simulink model "PI_5-67"  (R2025a)
settings: Solver=VariableStepAuto  StartTime=0.0  StopTime=10.0  RelTol=1e-3
values from neighbouring files (symbols this model uses):
  alpha = a    (= 20.6731)    [Rocky_5_closed_loop_poles.m]    (also in Rocky_67.m = a; pole5.m = a)
  beta = b    (= 0.001719)    [Rocky_5_closed_loop_poles.m]    (also in Rocky_67.m = b; pole5.m = b)
  dist_duration = .1    (= 0.1)    [Rocky_5_closed_loop_poles.m]    (also in Rocky_67.m; pole5.m)
  dist_magnitude = pi()/18    [Rocky_5_closed_loop_poles.m]    (also in Rocky_67.m; pole5.m)
  dist_time = 1    [Rocky_5_closed_loop_poles.m]    (also in Rocky_67.m; pole5.m)
  Ki = double(solutions.Ki)    [Rocky_5_closed_loop_poles.m]    (also in Rocky_67.m = (leff / (alpha * beta)) * (alpha^3 / 27 + alpha * omega_n^2); Rocky_closed_loop_poles_23.m; pole5.m = 16528)
  Kp = double(solutions.Kp)    [Rocky_5_closed_loop_poles.m]    (also in Rocky_67.m = (leff / (alpha * beta)) * (alpha^2 / 3 + omega_n^2); Rocky_closed_loop_poles_23.m; pole5.m = 3507.2)
  leff = l    (= 0.4452)    [Rocky_5_closed_loop_poles.m]    (also in Rocky_67.m = L; pole5.m = l)
  omega_n = 4.6939    [Rocky_5_closed_loop_poles.m]    (also in Rocky_67.m = omega_d / sqrt(1 - zeta^2); pole5.m)
  theta_r = 0    [Rocky_5_closed_loop_poles.m]    (also in Rocky_67.m; pole5.m)
libraries: slpidlib x1
settings Model: Creator=nbanse  LastModifiedBy=nbanse

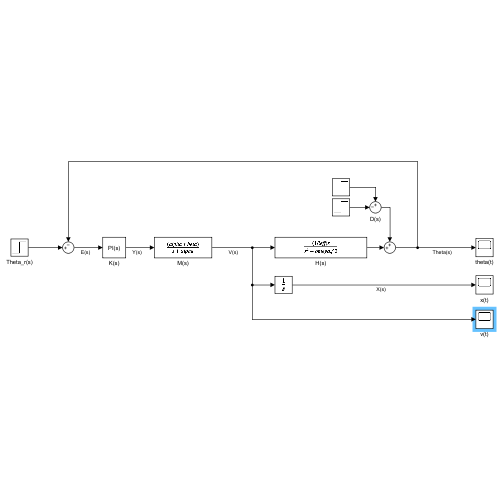
[thumbnail: Simulink's stored preview of the top-level diagram]
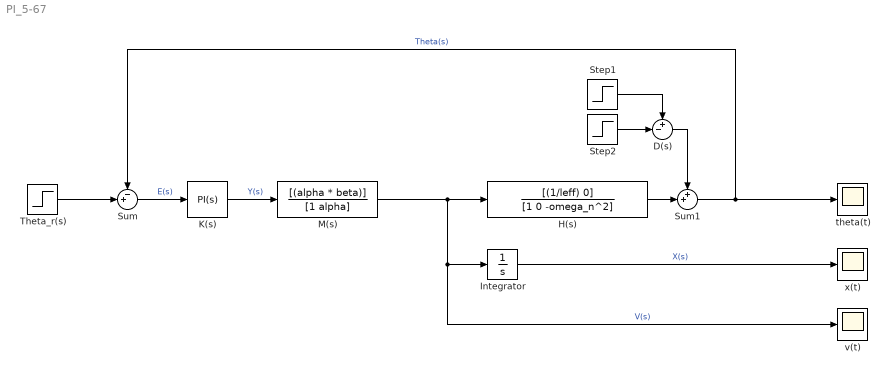
== system PI_5-67 ==
  D(s) : Sum  Inputs=+-|
  H(s) : TransferFcn  Numerator=[(1/leff) 0]  Denominator=[1 0 -omega_n^2]
  Integrator : Integrator
  K(s) : slpidlib/PID Controller  Controller=PI  Form=Parallel  TimeDomain=Continuous-time  UseExternalTs=off  SampleTime=-1  IntegratorMethod=Forward Euler  FilterMethod=Forward Euler  ControllerParametersSource=internal  P=Kp  I=Ki  UseKiTs=off  D=0  UseExternalDerivativeSource=off  N=100  UseFilter=on  TunerSelectOption=Transfer Function Based (PID Tuner App)  InitialConditionSource=internal  InitialConditionForIntegrator=0  InitialConditionForFilter=0  DifferentiatorICPrevScaledInput=0  ExternalReset=none  TrackingMode=off  Kt=1  LimitOutput=off  SatLimitsSource=internal  UpperSaturationLimit=inf  LowerSaturationLimit=-inf  LinearizeAsGain=on  AntiWindupMode=none  Kb=1  LimitIntegrator=off  UpperIntegratorSaturationLimit=inf  LowerIntegratorSaturationLimit=-inf  POutMin=[]  POutMax=[]  IOutMin=[]  IOutMax=[]  DOutMin=[]  DOutMax=[]  NOutMin=[]  NOutMax=[]  SumOutMin=[]  SumOutMax=[]  SaturationOutMin=[]  SaturationOutMax=[]  PParamMin=[]  PParamMax=[]  IParamMin=[]  IParamMax=[]  DParamMin=[]  DParamMax=[]  NParamMin=[]  NParamMax=[]  KbParamMin=[]  KbParamMax=[]  KtParamMin=[]  KtParamMax=[]  KbOutMin=[]  KbOutMax=[]  KtOutMin=[]  KtOutMax=[]  IntegratorOutMin=[]  IntegratorOutMax=[]  FilterOutMin=[]  FilterOutMax=[]  SumI1OutMin=[]  SumI1OutMax=[]  SumI2OutMin=[]  SumI2OutMax=[]  SumI3OutMin=[]  SumI3OutMax=[]  SumI4OutMin=[]  SumI4OutMax=[]  SumDOutMin=[]  SumDOutMax=[]  DifferentiatorOutMin=[]  DifferentiatorOutMax=[]  FilterDiffOutCoefMin=[]  FilterDiffOutCoefMax=[]  ReciprocalOutMin=[]  ReciprocalOutMax=[]  SumDenOutMin=[]  SumDenOutMax=[]  SumNumOutMin=[]  SumNumOutMax=[]  DivideOutMin=[]  DivideOutMax=[]  UdiffTsProdOutMin=[]  UdiffTsProdOutMax=[]  NTsProdOutMin=[]  NTsProdOutMax=[]  UintegralTsProdOutMin=[]  UintegralTsProdOutMax=[]  UngainTsProdOutMin=[]  UngainTsProdOutMax=[]  ClampingZeroOutDataTypeStr=Inherit: Inherit via back propagation  ClampingZeroOutMin=[]  ClampingZeroOutMax=[]  FilterDenConstantOutDataTypeStr=Inherit: Inherit via back propagation  FilterDenConstantOutMin=[]  FilterDenConstantOutMax=[]  PCopyOutDataTypeStr=Inherit: Inherit via back propagation  PCopyOutMin=[]  PCopyOutMax=[]  NCopyOutDataTypeStr=Inherit: Inherit via back propagation  NCopyOutMin=[]  NCopyOutMax=[]  IntegratorContinuousStateAttributes=''  IntegratorStateMustResolveToSignalObject=off  IntegratorRTWStateStorageClass=Auto  FilterContinuousStateAttributes=''  FilterStateMustResolveToSignalObject=off  FilterRTWStateStorageClass=Auto  ParallelPVariant=InternalParameters  IdealPVariant=Disabled  IVariant=InternalParameters  DVariant=Disabled  IntegratorVariant=Continuous  SatVariant=Disabled  AWVariant=Passthrough  PCopyVariant=Disabled  TRVariant=Disabled  FdbkBlocksVariant=Forward  IdealPFdbkVariant=Disabled  SatFdbkVariant=Disabled  DerivativeFilterVariant=Disabled  NVariant=Disabled  NCopyVariant=Disabled_SignalSpec  FilterICVariant=Disabled  IntegratorICVariant=InternalICs  ExternalResetVariant=Disabled  TRSumVariant=Passthrough  SumFdbkVariant=Disabled  SumVariant=Sum_PI  TsampFilterVariant=InternalTs  TsampNgainVariant=Passthrough  TsampIntegralVariant=Disabled_SignalSpec  ExternalSaturationOutDataTypeStr=Inherit: Same as second input  DerivativeSourceVariant=Disabled  PreIntVariant=InternalPreInt
  M(s) : TransferFcn  Numerator=[(alpha * beta)]  Denominator=[1 alpha]
  Step1 : Step  Time=dist_time  After=dist_magnitude  SampleTime=0
  Step2 : Step  Time=dist_time+dist_duration  After=dist_magnitude  SampleTime=0
  Sum : Sum  Inputs=-+|
  Sum1 : Sum  Inputs=++|
  Theta_r(s) : Step  Time=0  After=theta_r  SampleTime=0
  theta(t) : Scope
      settings: ActiveDisplayYMinimum=-0.18045981547498627  ActiveDisplayYMaximum=0.21397656305214618
  v(t) : Scope
      settings: ActiveDisplayYMinimum=-0.765089378525378  ActiveDisplayYMaximum=0.65342094207672474  DataLoggingVariableName=ScopeData2
  x(t) : Scope
      settings: ActiveDisplayYMinimum=-0.41604003873101825  ActiveDisplayYMaximum=3.1542227118533162
  wires:
  H(s)/1 -> Sum1/2
  M(s)/1 -> H(s)/1, Integrator/1, v(t)/1  "V(s)"
  Step1/1 -> D(s)/1
  Step2/1 -> D(s)/2
  K(s)/1 -> M(s)/1  "Y(s)"
  Sum/1 -> K(s)/1  "E(s)"
  D(s)/1 -> Sum1/1
  Sum1/1 -> Sum/1, theta(t)/1  "Theta(s)"
  Theta_r(s)/1 -> Sum/2
  Integrator/1 -> x(t)/1  "X(s)"
